simulink model "SIMULACION_TORQUE"  (Simulink 7.7)
settings: Solver=ode2  StartTime=0.0  StopTime=inf  RelTol=1e-3
libraries: simulink x4
settings Model: Creator=JohnConstantine  LastModifiedBy=JohnConstantine

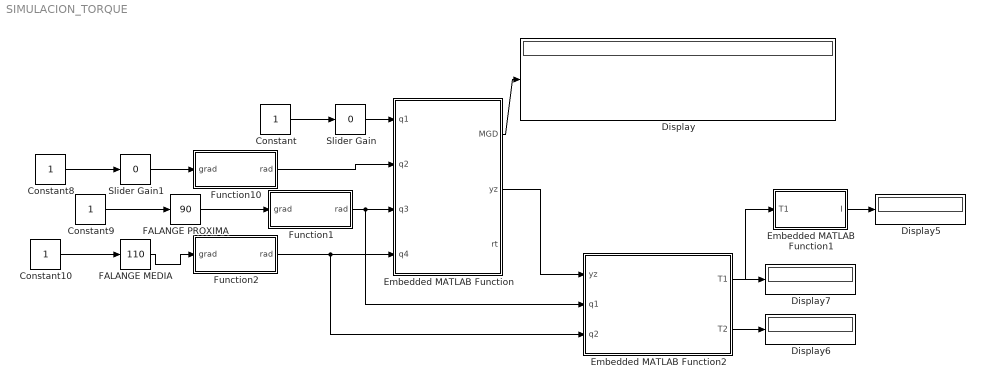
== system SIMULACION_TORQUE ==
  Constant{,8..10} (4 alike) : Constant
  Display{,5..7} (4 alike) : Display
  Embedded MATLAB Function : Stateflow chart  TreatAsAtomicUnit=on
  Embedded MATLAB Function1 : Stateflow chart  TreatAsAtomicUnit=on
  Embedded MATLAB Function2 : Stateflow chart  TreatAsAtomicUnit=on
  FALANGE MEDIA : simulink/Math Operations/Slider Gain  SystemSampleTime=-1  low=0  gain=110  high=110
  FALANGE PROXIMA : simulink/Math Operations/Slider Gain  SystemSampleTime=-1  low=0  gain=90  high=90
  Function1 : Stateflow chart  TreatAsAtomicUnit=on
  Function10 : Stateflow chart  TreatAsAtomicUnit=on
  Function2 : Stateflow chart  TreatAsAtomicUnit=on
  Slider Gain : simulink/Math Operations/Slider Gain  SystemSampleTime=-1  low=0  gain=0  high=2.5
  Slider Gain1 : simulink/Math Operations/Slider Gain  SystemSampleTime=-1  low=0  gain=0  high=15
  wires:
  Constant/1 -> Slider Gain/1
  Constant8/1 -> Slider Gain1/1
  Constant9/1 -> FALANGE PROXIMA/1
  Constant10/1 -> FALANGE MEDIA/1
  Function10/1(rad) -> Embedded MATLAB Function/2(q2)
  Slider Gain1/1 -> Function10/1(grad)
  FALANGE PROXIMA/1 -> Function1/1(grad)
  Function1/1(rad) -> Embedded MATLAB Function/3(q3), Embedded MATLAB Function2/2(q1)
  Function2/1(rad) -> Embedded MATLAB Function/4(q4), Embedded MATLAB Function2/3(q2)
  FALANGE MEDIA/1 -> Function2/1(grad)
  Slider Gain/1 -> Embedded MATLAB Function/1(q1)
  Embedded MATLAB Function/1(MGD) -> Display/1
  Embedded MATLAB Function2/1(T1) -> Display7/1, Embedded MATLAB Function1/1(T1)
  Embedded MATLAB Function2/2(T2) -> Display6/1
  Embedded MATLAB Function/2(yz) -> Embedded MATLAB Function2/1(yz)
  Embedded MATLAB Function1/1(I) -> Display5/1

== matlab function Function1 ==
  data: grad input double; rad output double
function rad =grad2rad(grad)

rad=grad*2*pi/360;

%d2r=pi/180;

== matlab function Embedded MATLAB Function ==
  data: q1 input double; MGD output double; q2 input double; q3 input double; q4 input double; yz output double; rt output double
function [MGD,yz,rt] =mgdFalange(q1,q2,q3,q4)

d2=0;
a2=.9907;
a3=.8862;
a4=1.5;
a5=.59;
a6=.59;

 MGD=[ -cos(q3 + q4)*sin(q2),  sin(q3 + q4)*sin(q2), cos(q2),                                         -sin(q2)*(a2 + a5*cos(q3 + q4) + a6*cos(q3 + q4) + a3*cos(q3) + a4*cos(q3));...
               -sin(q3 + q4),         -cos(q3 + q4),       0,                                                  - d2 - a5*sin(q3 + q4) - a6*sin(q3 + q4) - a3*sin(q3) - a4*sin(q3);...
        cos(q3 + q4)*cos(q2), -sin(q3 + q4)*cos(q2), sin(q2), q1 + a2*cos(q2) + cos(q2)*cos(q3)*(a3 + a4) - cos(q2)*sin(q3)*sin(q4)*(a5 + a6) + cos(q2)*cos(q3)*cos(q4)*(a5 + a6);...
                           0,                     0,       0,                                                                                                                  1];
                                                                                                                                                                                                                                                                                 
H=MGD;
yz=[MGD(2,4) MGD(3,4)];


% r21=H(2,1);
% r11=H(1,1);
% r31=H(3,1);
% r32=H(3,2);
% r33=H(3,3);



rt=[H(2,1) H(1,1) H(3,1) H(3,2) H(3,3);];%Las posiciones de la matriz de rotacion de los angulos de EULER y RPY para el calculo de alpha, gamma, theta

== matlab function Function2 ==
  data: grad input double; rad output double
function rad =grad2rad(grad)

rad=grad*2*pi/360;

== matlab function Embedded MATLAB Function1 ==
  data: T1 input double; I output double
function I =Current(T1)

%T1=T(1);
%T2=T(2);

K=0.01; %Nm/Amp

I=T1/K;

== matlab function Embedded MATLAB Function2 ==
  data: yz input double; T1 output double; T2 output double; q1 input double; q2 input double
function [T1,T2]  =Torque(yz,q1,q2)
y=abs(yz(1));
z=abs(yz(2));

r1=2.3862;
r2=sqrt(y^2+z^2);
r3=.59+.59;

B=atan(y/z);

f1=3.9;%N
f2=3.2;%N

 T1=(r1*f1*sin(q1))+(r2*f2*sin(B));
 T2=(r3*f2*sin(q2));

== matlab function Function10 ==
  data: grad input double; rad output double
function rad =grad2rad(grad)

rad=grad*2*pi/360;
